simulink model "Exercicios_1_2_3"  (R2015b)
settings: Solver=VariableStepAuto  StartTime=0.0  StopTime=1.5  RelTol=1e-3
libraries: simulink x1
settings Model: Creator=aluno  LastModifiedBy=aluno

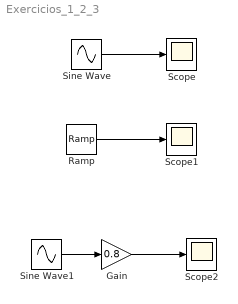
== system Exercicios_1_2_3 ==
  Gain : Gain  Gain=0.8
  Ramp : simulink/Sources/Ramp  slope=3  start=0  X0=0
  Scope : Scope
  Scope1 : Scope
  Scope2 : Scope
  Sine Wave : Sin  Amplitude=4.55  Frequency=12.56  SampleTime=0
  Sine Wave1 : Sin  Amplitude=2  Frequency=6.28  SampleTime=0
  wires:
  Sine Wave/1 -> Scope/1
  Ramp/1 -> Scope1/1
  Sine Wave1/1 -> Gain/1
  Gain/1 -> Scope2/1
